simulink model "gm_sampleModel1519_sub_sub_sub"  (R2023a)
settings: Solver=VariableStepAuto  StartTime=0.0  StopTime=10.0  RelTol=1e-3
libraries: simulink x2, hdlsllib x2
settings Model: Creator=user1  LastModifiedBy=user1
settings OptimizationCC: BlockReduction=off  ConditionallyExecuteInputs=off
settings DebuggingCC: InheritedTsInSrcMsg=none

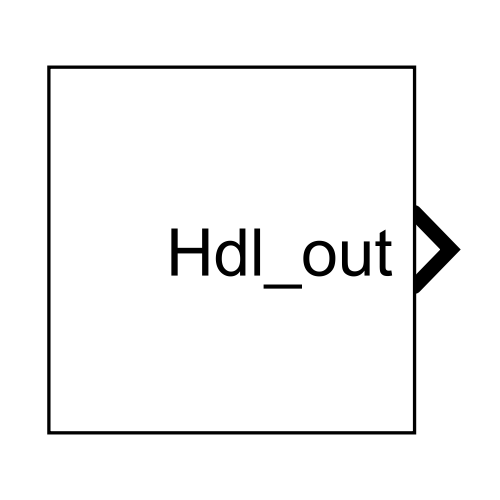
[thumbnail: Simulink's stored preview of the top-level diagram]
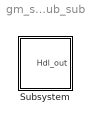
== system gm_sampleModel1519_sub_sub_sub ==
  Subsystem : Subsystem

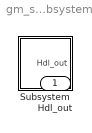
== system gm_sampleModel1519_sub_sub_sub/Subsystem ==
  Subsystem : Subsystem
  Hdl_out : Outport  OutDataTypeStr=uint8

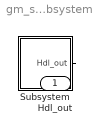
== system gm_sampleModel1519_sub_sub_sub/Subsystem/Subsystem ==
  Subsystem : Subsystem
  Hdl_out : Outport  OutDataTypeStr=uint8
  wires:
  Subsystem/1(Hdl_out) -> Hdl_out/1

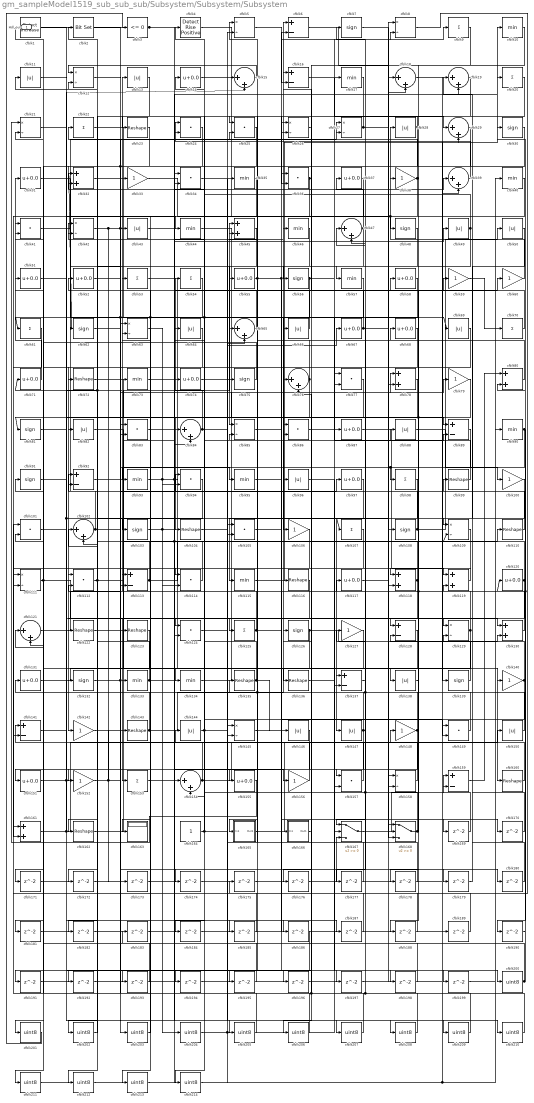
== system gm_sampleModel1519_sub_sub_sub/Subsystem/Subsystem/Subsystem ==
  cfblk1 : simulink/Logic and Bit Operations/Detect Increase  vinit=0.0  OutDataTypeStr=uint8
      settings: LibrarySourceBlock=|
      | hdlsllib/Logic and Bit
      | Operations/Detect
      | Increase
  cfblk{10,17,35,40,44,46,57,73,90,93,95,115,133..134} (14 alike) : MinMax  OutDataTypeStr=uint8
  cfblk{33,38,59..60,79,100,106,127,140,142,148,152,156} (13 alike) : Gain  OutDataTypeStr=uint8
  cfblk{24..25,34,36,41,77,83,86,94,101,105,112,114,124,149,157} (16 alike) : DotProduct  OutDataTypeStr=uint8
  cfblk{15,18..19,29,39,47,65,76,84,102,121,154} (12 alike) : Sum  Inputs=|++  OutDataTypeStr=uint8
  cfblk{7,30,48,56,62,75,81,91,103,108,126,132,139} (13 alike) : Signum
  cfblk{23,72,99,104,110,116,122..123,135..136,143,160,162} (13 alike) : Reshape
  cfblk{9,20,22,53..54,61,70,98,107,125,153} (11 alike) : Sum  Inputs=+  OutDataTypeStr=uint8
  cfblk{5,8,12,21,26..27,42,63,85,109,111,129,145,158} (14 alike) : Product  Inputs=*/  OutDataTypeStr=uint8  RndMeth=Zero  SaturateOnIntegerOverflow=on
  cfblk{11,13,28,43,49..50,64,66,69,82,88,96,138,144,146..147,150} (17 alike) : Abs  OutDataTypeStr=uint8  SaturateOnIntegerOverflow=off
  cfblk{6,16,89,92,113,128,137,141,159} (9 alike) : Sum  Inputs=+-  OutDataTypeStr=uint8
  cfblk{14,31,37,51..52,55,58,67..68,71,74,87,97,117,120,131,151,155} (18 alike) : Bias  Bias=0.0  SaturateOnIntegerOverflow=off
  cfblk{32,45,78,80,118..119,130,161} (8 alike) : Sum  OutDataTypeStr=uint8
  cfblk163 : Display
  cfblk164 : Constant  OutDataTypeStr=uint8  SampleTime=-1
  cfblk165 : Subsystem
      settings: LibrarySourceBlock=|
      | hdlsllib/Ports &
      | Subsystems/Subsystem
  cfblk166 : Subsystem
      settings: LibrarySourceBlock=|
      | hdlsllib/Ports &
      | Subsystems/Subsystem
  cfblk167 : Switch  OutDataTypeStr=uint8  SaturateOnIntegerOverflow=off  InputSameDT=off
  cfblk168 : Switch  OutDataTypeStr=uint8  SaturateOnIntegerOverflow=off  InputSameDT=off
  cfblk{169..199} (31 alike) : Delay  SampleTime=1
  cfblk2 : simulink/Logic and Bit Operations/Bit Set  iBit=0
      settings: LibrarySourceBlock=|
      | hdlsllib/Logic and Bit
      | Operations/Bit Set
  cfblk{200..214} (15 alike) : DataTypeConversion  OutDataTypeStr=uint8  SaturateOnIntegerOverflow=off  RndMeth=Floor
  cfblk3 : hdlsllib/Logic and Bit Operations/Compare To Zero  relop=<=  OutDataTypeStr=uint8
  cfblk4 : hdlsllib/Logic and Bit Operations/Detect Rise Positive  vinit=0  OutDataTypeStr=uint8
  Hdl_out : Outport  OutDataTypeStr=uint8
  wires:
  cfblk214/1 -> cfblk35/1
  cfblk213/1 -> cfblk189/1, cfblk90/1
  cfblk212/1 -> cfblk34/2
  cfblk211/1 -> cfblk34/1
  cfblk186/1 -> cfblk211/1
  cfblk210/1 -> cfblk86/2, cfblk111/1, cfblk47/1
  cfblk209/1 -> cfblk101/2
  cfblk208/1 -> cfblk101/1
  cfblk73/1 -> cfblk208/1
  cfblk207/1 -> cfblk91/1
  cfblk101/1 -> cfblk207/1
  cfblk206/1 -> cfblk63/2
  cfblk205/1 -> cfblk63/1
  cfblk182/1 -> cfblk205/1
  cfblk204/1 -> cfblk15/1, cfblk77/1
  cfblk203/1 -> cfblk183/1
  cfblk2/1 -> cfblk203/1
  cfblk202/1 -> cfblk2/1
  cfblk23/1 -> cfblk202/1
  cfblk201/1 -> cfblk3/1
  cfblk200/1 -> cfblk120/1, cfblk30/1, cfblk102/1
  cfblk199/1 -> cfblk40/1
  cfblk136/1 -> cfblk199/1
  cfblk198/1 -> cfblk167/2
  cfblk197/1 -> cfblk47/2
  cfblk196/1 -> cfblk149/1
  cfblk9/1 -> cfblk196/1
  cfblk195/1 -> cfblk1/1
  cfblk194/1 -> cfblk118/2
  cfblk141/1 -> cfblk194/1
  cfblk193/1 -> cfblk83/1
  cfblk192/1 -> cfblk124/2
  cfblk94/1 -> cfblk192/1
  cfblk191/1 -> cfblk154/1
  cfblk68/1 -> cfblk191/1
  cfblk190/1 -> cfblk80/2
  cfblk189/1 -> cfblk112/2
  cfblk188/1 -> cfblk121/1
  cfblk30/1 -> cfblk188/1
  cfblk187/1 -> cfblk36/1
  cfblk95/1 -> cfblk187/1
  cfblk91/1 -> cfblk186/1
  cfblk185/1 -> cfblk161/1
  cfblk11/1 -> cfblk185/1
  cfblk184/1 -> cfblk39/2
  cfblk183/1 -> cfblk77/2
  cfblk109/1 -> cfblk182/1
  cfblk181/1 -> cfblk26/1
  cfblk146/1 -> cfblk181/1
  cfblk180/1 -> cfblk129/2
  cfblk142/1 -> cfblk180/1
  cfblk179/1 -> cfblk119/2
  cfblk178/1 -> cfblk45/2
  cfblk177/1 -> cfblk105/1
  cfblk128/1 -> cfblk177/1
  cfblk176/1 -> cfblk29/2
  cfblk175/1 -> cfblk18/1
  cfblk8/1 -> cfblk175/1
  cfblk174/1 -> cfblk5/2
  cfblk173/1 -> cfblk6/2
  cfblk172/1 -> cfblk65/2
  cfblk116/1 -> cfblk172/1
  cfblk171/1 -> cfblk167/3
  cfblk170/1 -> cfblk19/1
  cfblk96/1 -> cfblk170/1
  cfblk169/1 -> cfblk159/2
  cfblk145/1 -> cfblk169/1
  cfblk85/1 -> cfblk116/1
  cfblk166/1(Out1) -> cfblk86/1
  cfblk160/1 -> cfblk141/1
  cfblk72/1 -> cfblk166/1(In1)
  cfblk80/1 -> cfblk66/1
  cfblk112/1 -> cfblk84/2, cfblk212/1
  cfblk61/1 -> cfblk161/2
  cfblk90/1 -> cfblk98/1, cfblk163/1, cfblk190/1
  cfblk103/1 -> cfblk109/2, cfblk156/1, cfblk114/2
  cfblk147/1 -> cfblk51/1, cfblk85/2, cfblk7/1, cfblk171/1
  cfblk158/1 -> cfblk135/1
  cfblk55/1 -> cfblk9/1, cfblk197/1, cfblk195/1
  cfblk154/1 -> cfblk26/2, cfblk113/1
  cfblk36/1 -> cfblk76/1, cfblk102/2
  cfblk67/1 -> cfblk59/1, cfblk42/2
  cfblk27/1 -> cfblk158/2, cfblk25/1
  cfblk29/1 -> cfblk121/2
  cfblk133/1 -> cfblk49/1, cfblk92/2
  cfblk92/1 -> cfblk60/1
  cfblk157/1 -> cfblk126/1
  cfblk135/1 -> cfblk64/1, cfblk146/1
  cfblk7/1 -> cfblk168/2
  cfblk35/1 -> cfblk213/1
  cfblk120/1 -> cfblk157/2, cfblk94/1
  cfblk89/1 -> cfblk145/2
  cfblk14/1 -> cfblk168/1
  cfblk86/1 -> cfblk89/2
  cfblk50/1 -> cfblk109/1
  cfblk45/1 -> cfblk152/1
  cfblk150/1 -> cfblk41/2, cfblk27/2
  cfblk153/1 -> cfblk46/1
  cfblk79/1 -> cfblk81/1, cfblk178/1
  cfblk15/1 -> cfblk12/1
  cfblk138/1 -> cfblk68/1
  cfblk99/1 -> cfblk32/2
  cfblk140/1 -> cfblk154/2, cfblk99/1
  cfblk3/1 -> cfblk200/1, Hdl_out/1
  cfblk18/1 -> cfblk140/1
  cfblk165/1(Out1) -> cfblk148/1
  cfblk104/1 -> cfblk145/1
  cfblk81/1 -> cfblk107/1, cfblk128/1
  cfblk47/1 -> cfblk57/1, cfblk37/1
  cfblk33/1 -> cfblk108/1
  cfblk46/1 -> cfblk105/2
  cfblk75/1 -> cfblk41/1
  cfblk41/1 -> cfblk123/1
  cfblk132/1 -> cfblk79/1, cfblk179/1
  cfblk137/1 -> cfblk157/1
  cfblk12/1 -> cfblk69/1, cfblk137/2
  cfblk32/1 -> cfblk43/1, cfblk95/1
  cfblk93/1 -> cfblk168/3, cfblk198/1, cfblk94/2
  cfblk51/1 -> cfblk89/1
  cfblk83/1 -> cfblk20/1
  cfblk148/1 -> cfblk117/1, cfblk176/1
  cfblk28/1 -> cfblk23/1, cfblk184/1
  cfblk113/1 -> cfblk11/1, cfblk78/2
  cfblk78/1 -> cfblk122/1
  cfblk52/1 -> cfblk129/1
  cfblk114/1 -> cfblk53/1
  cfblk123/1 -> cfblk132/1
  cfblk40/1 -> cfblk136/1
  cfblk156/1 -> cfblk74/1
  cfblk121/1 -> cfblk83/2
  cfblk58/1 -> cfblk167/1
  cfblk152/1 -> cfblk96/1, cfblk143/1
  cfblk124/1 -> cfblk38/1
  cfblk62/1 -> cfblk33/1
  cfblk19/1 -> cfblk65/1
  cfblk77/1 -> cfblk112/1
  cfblk37/1 -> cfblk103/1
  cfblk60/1 -> cfblk28/1
  cfblk24/1 -> cfblk162/1
  cfblk164/1 -> cfblk144/1, cfblk110/1
  cfblk21/1 -> cfblk84/1
  cfblk26/1 -> cfblk56/1
  cfblk105/1 -> cfblk149/2
  cfblk54/1 -> cfblk82/1
  cfblk20/1 -> cfblk124/1
  cfblk100/1 -> cfblk125/1
  cfblk57/1 -> cfblk114/1, cfblk193/1
  cfblk84/1 -> cfblk54/1, cfblk209/1
  cfblk130/1 -> cfblk32/1
  cfblk126/1 -> cfblk130/2, cfblk214/1
  cfblk43/1 -> cfblk39/1
  cfblk129/1 -> cfblk88/1, cfblk76/2, cfblk155/1
  cfblk5/1 -> cfblk16/2
  cfblk56/1 -> cfblk61/1, cfblk93/1, cfblk8/2
  cfblk110/1 -> cfblk24/2
  cfblk17/1 -> cfblk36/2
  cfblk70/1 -> cfblk16/1
  cfblk76/1 -> cfblk104/1, cfblk5/1
  cfblk151/1 -> cfblk150/1, cfblk73/1
  cfblk16/1 -> cfblk29/1
  cfblk168/1 -> cfblk42/1, cfblk127/1, cfblk128/2
  cfblk6/1 -> cfblk18/2
  cfblk1/1 -> cfblk44/1
  cfblk122/1 -> cfblk75/1
  cfblk53/1 -> cfblk160/1
  cfblk117/1 -> cfblk8/1
  cfblk22/1 -> cfblk87/1
  cfblk131/1 -> cfblk133/1
  cfblk88/1 -> cfblk100/1
  cfblk161/1 -> cfblk17/1, cfblk15/2
  cfblk49/1 -> cfblk4/1, cfblk206/1
  cfblk167/1 -> cfblk159/1
  cfblk106/1 -> cfblk111/2
  cfblk66/1 -> cfblk52/1
  cfblk111/1 -> cfblk130/1, cfblk201/1
  cfblk4/1 -> cfblk158/1
  cfblk10/1 -> cfblk138/1
  cfblk144/1 -> cfblk14/1, cfblk67/1
  cfblk13/1 -> cfblk72/1
  cfblk155/1 -> cfblk21/1
  cfblk74/1 -> cfblk55/1
  cfblk44/1 -> cfblk139/1
  cfblk69/1 -> cfblk137/1
  cfblk39/1 -> cfblk24/1
  cfblk42/1 -> cfblk173/1, cfblk174/1
  cfblk64/1 -> cfblk142/1
  cfblk118/1 -> cfblk12/2, cfblk71/1, cfblk153/1
  cfblk63/1 -> cfblk204/1
  cfblk65/1 -> cfblk45/1
  cfblk119/1 -> cfblk118/1
  cfblk107/1 -> cfblk165/1(In1)
  cfblk48/1 -> cfblk85/1
  cfblk31/1 -> cfblk106/1
  cfblk87/1 -> cfblk119/1
  cfblk98/1 -> cfblk115/1
  cfblk162/1 -> cfblk97/1
  cfblk108/1 -> cfblk50/1, cfblk92/1
  cfblk25/1 -> cfblk62/1, cfblk113/2
  cfblk139/1 -> cfblk58/1
  cfblk59/1 -> cfblk70/1
  cfblk134/1 -> cfblk78/1
  cfblk125/1 -> cfblk13/1, cfblk19/2
  cfblk159/1 -> cfblk80/1
  cfblk143/1 -> cfblk6/1, cfblk21/2
  cfblk127/1 -> cfblk151/1
  cfblk38/1 -> cfblk141/2, cfblk48/1, cfblk22/1
  cfblk34/1 -> cfblk210/1
  cfblk97/1 -> cfblk147/1
  cfblk115/1 -> cfblk10/1
  cfblk102/1 -> cfblk27/1, cfblk25/2
  cfblk149/1 -> cfblk131/1
  cfblk82/1 -> cfblk134/1
  cfblk71/1 -> cfblk31/1

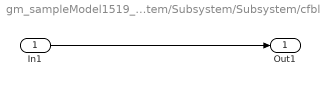
== system gm_sampleModel1519_sub_sub_sub/Subsystem/Subsystem/Subsystem/cfblk165 ==
  In1 : Inport
  Out1 : Outport
  wires:
  In1/1 -> Out1/1

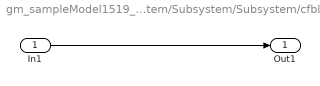
== system gm_sampleModel1519_sub_sub_sub/Subsystem/Subsystem/Subsystem/cfblk166 ==
  In1 : Inport
  Out1 : Outport
  wires:
  In1/1 -> Out1/1
